simulink model "collision"  (R2018a)
settings: Solver=VariableStepAuto  StartTime=0.0  StopTime=120  FixedStep=0.01  MaxStep=.01  RelTol=1e-3
settings Model: Creator=U500304  LastModifiedBy=U500304
settings SolverCC: ZeroCrossAlgorithm=Adaptive
settings DataIOCC: SaveOutput=off  SaveTime=off
settings DebuggingCC: MaxConsecutiveZCsMsg=warning

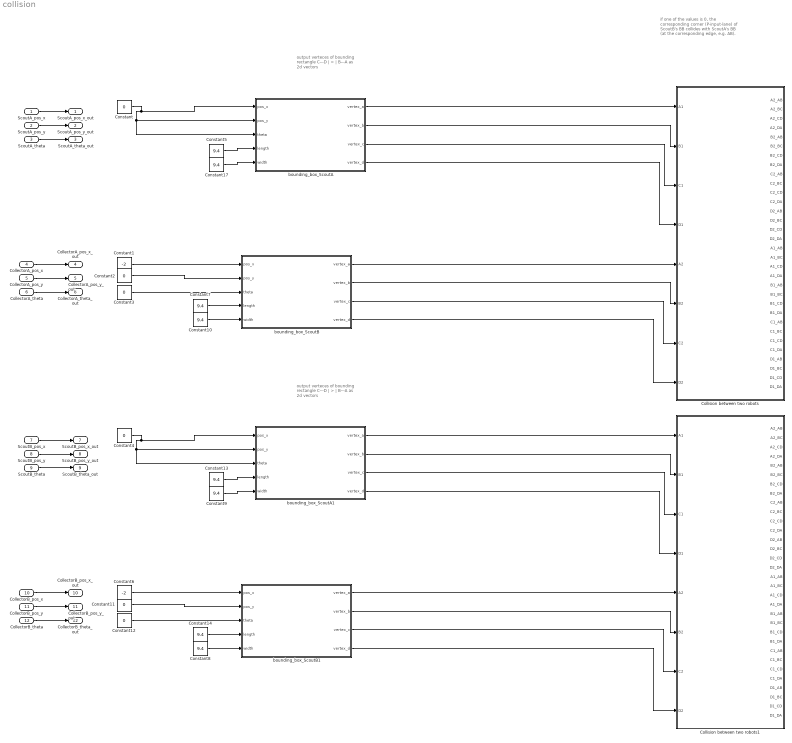
== system collision ==
  note: if one of the values is 0, the corresponding corner (P-input-lane) of ScoutB's BB collides with ScoutA's BB (at the corresponding edge, e.g. AB).
  note: output verteces of
      | bounding rectangle
      | C---D
      | |  >  |
      | B---A  as 2d vectors
  note: output verteces of
      | bounding rectangle
      | C---D
      | |  >  |
      | B---A  as 2d vectors
  ScoutA_pos_x : Inport  OutDataTypeStr=double  PortDimensions=1  SampleTime=0
  ScoutA_pos_y : Inport  Port=2  OutDataTypeStr=double  PortDimensions=1  SampleTime=0
  ScoutA_theta : Inport  Port=3  OutDataTypeStr=double  PortDimensions=1  SampleTime=0
  CollectorA_pos_x : Inport  Port=4  OutDataTypeStr=double  PortDimensions=1  SampleTime=0
  CollectorA_pos_y : Inport  Port=5  OutDataTypeStr=double  PortDimensions=1  SampleTime=0
  CollectorA_theta : Inport  Port=6  OutDataTypeStr=double  PortDimensions=1  SampleTime=0
  ScoutB_pos_x : Inport  Port=7  OutDataTypeStr=double  PortDimensions=1  SampleTime=0
  ScoutB_pos_y : Inport  Port=8  OutDataTypeStr=double  PortDimensions=1  SampleTime=0
  ScoutB_theta : Inport  Port=9  OutDataTypeStr=double  PortDimensions=1  SampleTime=0
  CollectorB_pos_x : Inport  Port=10  OutDataTypeStr=double  PortDimensions=1  SampleTime=0
  CollectorB_pos_y : Inport  Port=11  OutDataTypeStr=double  PortDimensions=1  SampleTime=0
  CollectorB_theta : Inport  Port=12  OutDataTypeStr=double  PortDimensions=1  SampleTime=0
  Collision between two robots : Subsystem
  Collision between two robots1 : Subsystem
  Constant{,2..4,11..12} (6 alike) : Constant  Value=0
  Constant1 : Constant  Value=-2
  Constant{5,7..10,13..14,17} (8 alike) : Constant  Value=9.4
  Constant6 : Constant  Value=-2
  bounding_box_ScoutA : Subsystem
  bounding_box_ScoutA1 : Subsystem
  bounding_box_ScoutB : Subsystem
  bounding_box_ScoutB1 : Subsystem
  ScoutA_pos_x_out : Outport
  ScoutA_pos_y_out : Outport  Port=2
  ScoutA_theta_out : Outport  Port=3
  CollectorA_pos_x_out : Outport  Port=4
  CollectorA_pos_y_out : Outport  Port=5
  CollectorA_theta_out : Outport  Port=6
  ScoutB_pos_x_out : Outport  Port=7
  ScoutB_pos_y_out : Outport  Port=8
  ScoutB_theta_out : Outport  Port=9
  CollectorB_pos_x_out : Outport  Port=10
  CollectorB_pos_y_out : Outport  Port=11
  CollectorB_theta_out : Outport  Port=12
  wires:
  Constant10/1 -> bounding_box_ScoutB/5(width)
  Constant17/1 -> bounding_box_ScoutA/5(width)
  Constant7/1 -> bounding_box_ScoutB/4(length)
  Constant3/1 -> bounding_box_ScoutB/3(theta)
  Constant5/1 -> bounding_box_ScoutA/4(length)
  Constant1/1 -> bounding_box_ScoutB/1(pos_x)
  Constant2/1 -> bounding_box_ScoutB/2(pos_y)
  Constant/1 -> bounding_box_ScoutA/3(theta), bounding_box_ScoutA/2(pos_y), bounding_box_ScoutA/1(pos_x)
  bounding_box_ScoutA/1(vertex_a) -> Collision between two robots/1(A1)
  bounding_box_ScoutA/2(vertex_b) -> Collision between two robots/2(B1)
  bounding_box_ScoutA/3(vertex_c) -> Collision between two robots/3(C1)
  bounding_box_ScoutA/4(vertex_d) -> Collision between two robots/4(D1)
  bounding_box_ScoutB/1(vertex_a) -> Collision between two robots/5(A2)
  bounding_box_ScoutB/2(vertex_b) -> Collision between two robots/6(B2)
  bounding_box_ScoutB/3(vertex_c) -> Collision between two robots/7(C2)
  bounding_box_ScoutB/4(vertex_d) -> Collision between two robots/8(D2)
  bounding_box_ScoutB1/4(vertex_d) -> Collision between two robots1/8(D2)
  bounding_box_ScoutB1/3(vertex_c) -> Collision between two robots1/7(C2)
  bounding_box_ScoutB1/2(vertex_b) -> Collision between two robots1/6(B2)
  bounding_box_ScoutB1/1(vertex_a) -> Collision between two robots1/5(A2)
  bounding_box_ScoutA1/4(vertex_d) -> Collision between two robots1/4(D1)
  bounding_box_ScoutA1/3(vertex_c) -> Collision between two robots1/3(C1)
  bounding_box_ScoutA1/2(vertex_b) -> Collision between two robots1/2(B1)
  bounding_box_ScoutA1/1(vertex_a) -> Collision between two robots1/1(A1)
  Constant4/1 -> bounding_box_ScoutA1/1(pos_x), bounding_box_ScoutA1/2(pos_y), bounding_box_ScoutA1/3(theta)
  Constant11/1 -> bounding_box_ScoutB1/2(pos_y)
  Constant6/1 -> bounding_box_ScoutB1/1(pos_x)
  Constant13/1 -> bounding_box_ScoutA1/4(length)
  Constant12/1 -> bounding_box_ScoutB1/3(theta)
  Constant14/1 -> bounding_box_ScoutB1/4(length)
  Constant9/1 -> bounding_box_ScoutA1/5(width)
  Constant8/1 -> bounding_box_ScoutB1/5(width)
  ScoutA_pos_x/1 -> ScoutA_pos_x_out/1
  ScoutA_pos_y/1 -> ScoutA_pos_y_out/1
  ScoutA_theta/1 -> ScoutA_theta_out/1
  CollectorA_pos_y/1 -> CollectorA_pos_y_out/1
  CollectorA_pos_x/1 -> CollectorA_pos_x_out/1
  CollectorA_theta/1 -> CollectorA_theta_out/1
  ScoutB_theta/1 -> ScoutB_theta_out/1
  ScoutB_pos_y/1 -> ScoutB_pos_y_out/1
  ScoutB_pos_x/1 -> ScoutB_pos_x_out/1
  CollectorB_theta/1 -> CollectorB_theta_out/1
  CollectorB_pos_y/1 -> CollectorB_pos_y_out/1
  CollectorB_pos_x/1 -> CollectorB_pos_x_out/1

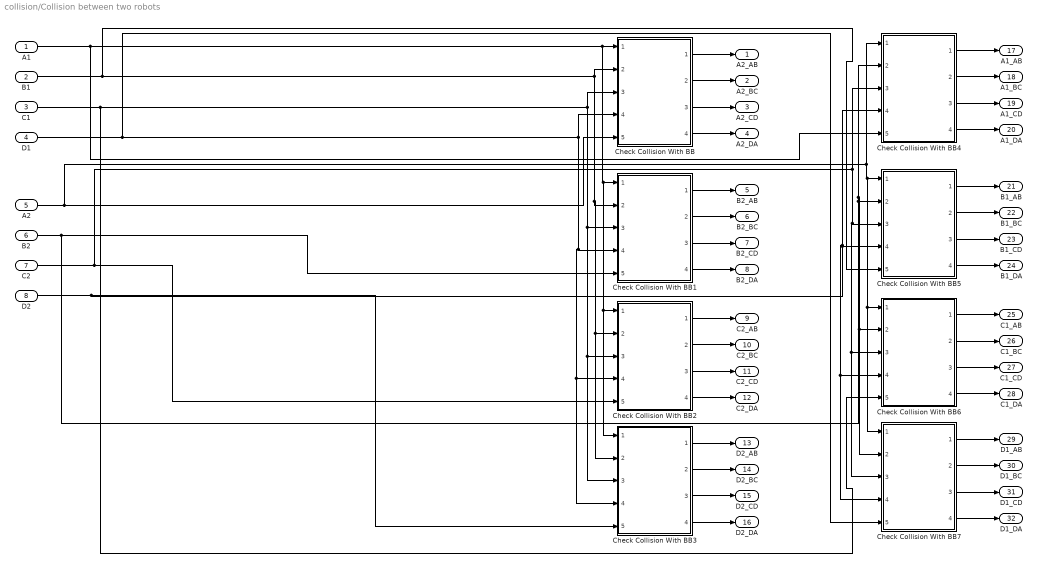
== system collision/Collision between two robots ==
  A1 : Inport
  B1 : Inport  Port=2
  C1 : Inport  Port=3
  D1 : Inport  Port=4
  A2 : Inport  Port=5
  B2 : Inport  Port=6
  C2 : Inport  Port=7
  D2 : Inport  Port=8
  Check Collision With BB{,1..7} (8 alike) : ModelReference  ModelNameDialog=check_collision_with_bounding  SimulationMode=Normal  ModelReferenceVersion=1.644
  A2_AB : Outport
  A2_BC : Outport  Port=2
  A2_CD : Outport  Port=3
  A2_DA : Outport  Port=4
  B2_AB : Outport  Port=5
  B2_BC : Outport  Port=6
  B2_CD : Outport  Port=7
  B2_DA : Outport  Port=8
  C2_AB : Outport  Port=9
  C2_BC : Outport  Port=10
  C2_CD : Outport  Port=11
  C2_DA : Outport  Port=12
  D2_AB : Outport  Port=13
  D2_BC : Outport  Port=14
  D2_CD : Outport  Port=15
  D2_DA : Outport  Port=16
  A1_AB : Outport  Port=17
  A1_BC : Outport  Port=18
  A1_CD : Outport  Port=19
  A1_DA : Outport  Port=20
  B1_AB : Outport  Port=21
  B1_BC : Outport  Port=22
  B1_CD : Outport  Port=23
  B1_DA : Outport  Port=24
  C1_AB : Outport  Port=25
  C1_BC : Outport  Port=26
  C1_CD : Outport  Port=27
  C1_DA : Outport  Port=28
  D1_AB : Outport  Port=29
  D1_BC : Outport  Port=30
  D1_CD : Outport  Port=31
  D1_DA : Outport  Port=32
  wires:
  Check Collision With BB3/3 -> D2_CD/1
  Check Collision With BB2/3 -> C2_CD/1
  Check Collision With BB/4 -> A2_DA/1
  Check Collision With BB/3 -> A2_CD/1
  Check Collision With BB1/3 -> B2_CD/1
  Check Collision With BB1/2 -> B2_BC/1
  Check Collision With BB2/1 -> C2_AB/1
  Check Collision With BB1/4 -> B2_DA/1
  Check Collision With BB/1 -> A2_AB/1
  Check Collision With BB1/1 -> B2_AB/1
  Check Collision With BB/2 -> A2_BC/1
  Check Collision With BB2/2 -> C2_BC/1
  Check Collision With BB3/4 -> D2_DA/1
  Check Collision With BB2/4 -> C2_DA/1
  Check Collision With BB3/1 -> D2_AB/1
  Check Collision With BB3/2 -> D2_BC/1
  Check Collision With BB6/3 -> C1_CD/1
  Check Collision With BB7/3 -> D1_CD/1
  Check Collision With BB7/1 -> D1_AB/1
  Check Collision With BB6/1 -> C1_AB/1
  Check Collision With BB7/4 -> D1_DA/1
  Check Collision With BB7/2 -> D1_BC/1
  Check Collision With BB4/4 -> A1_DA/1
  Check Collision With BB5/1 -> B1_AB/1
  Check Collision With BB5/4 -> B1_DA/1
  Check Collision With BB5/2 -> B1_BC/1
  Check Collision With BB4/3 -> A1_CD/1
  Check Collision With BB5/3 -> B1_CD/1
  D2/1 -> Check Collision With BB4/4, Check Collision With BB7/4, Check Collision With BB6/4, Check Collision With BB5/4, Check Collision With BB3/5
  Check Collision With BB4/1 -> A1_AB/1
  B2/1 -> Check Collision With BB4/2, Check Collision With BB7/2, Check Collision With BB6/2, Check Collision With BB5/2, Check Collision With BB1/5
  B1/1 -> Check Collision With BB5/5, Check Collision With BB/2, Check Collision With BB3/2, Check Collision With BB2/2, Check Collision With BB1/2
  C1/1 -> Check Collision With BB6/5, Check Collision With BB/3, Check Collision With BB3/3, Check Collision With BB2/3, Check Collision With BB1/3
  D1/1 -> Check Collision With BB7/5, Check Collision With BB/4, Check Collision With BB3/4, Check Collision With BB2/4, Check Collision With BB1/4
  C2/1 -> Check Collision With BB4/3, Check Collision With BB7/3, Check Collision With BB6/3, Check Collision With BB5/3, Check Collision With BB2/5
  Check Collision With BB6/2 -> C1_BC/1
  A2/1 -> Check Collision With BB4/1, Check Collision With BB7/1, Check Collision With BB6/1, Check Collision With BB5/1, Check Collision With BB/5
  Check Collision With BB4/2 -> A1_BC/1
  A1/1 -> Check Collision With BB4/5, Check Collision With BB/1, Check Collision With BB3/1, Check Collision With BB2/1, Check Collision With BB1/1
  Check Collision With BB6/4 -> C1_DA/1

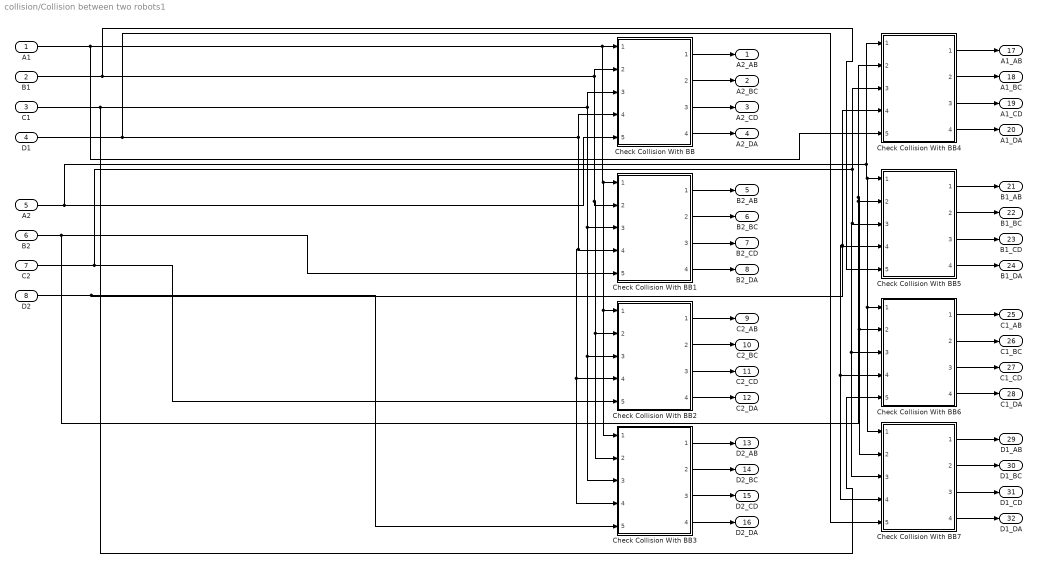
== system collision/Collision between two robots1 ==
  A1 : Inport
  B1 : Inport  Port=2
  C1 : Inport  Port=3
  D1 : Inport  Port=4
  A2 : Inport  Port=5
  B2 : Inport  Port=6
  C2 : Inport  Port=7
  D2 : Inport  Port=8
  Check Collision With BB{,1..7} (8 alike) : ModelReference  ModelNameDialog=check_collision_with_bounding  SimulationMode=Normal  ModelReferenceVersion=1.644
  A2_AB : Outport
  A2_BC : Outport  Port=2
  A2_CD : Outport  Port=3
  A2_DA : Outport  Port=4
  B2_AB : Outport  Port=5
  B2_BC : Outport  Port=6
  B2_CD : Outport  Port=7
  B2_DA : Outport  Port=8
  C2_AB : Outport  Port=9
  C2_BC : Outport  Port=10
  C2_CD : Outport  Port=11
  C2_DA : Outport  Port=12
  D2_AB : Outport  Port=13
  D2_BC : Outport  Port=14
  D2_CD : Outport  Port=15
  D2_DA : Outport  Port=16
  A1_AB : Outport  Port=17
  A1_BC : Outport  Port=18
  A1_CD : Outport  Port=19
  A1_DA : Outport  Port=20
  B1_AB : Outport  Port=21
  B1_BC : Outport  Port=22
  B1_CD : Outport  Port=23
  B1_DA : Outport  Port=24
  C1_AB : Outport  Port=25
  C1_BC : Outport  Port=26
  C1_CD : Outport  Port=27
  C1_DA : Outport  Port=28
  D1_AB : Outport  Port=29
  D1_BC : Outport  Port=30
  D1_CD : Outport  Port=31
  D1_DA : Outport  Port=32
  wires:
  Check Collision With BB6/4 -> C1_DA/1
  A1/1 -> Check Collision With BB1/1, Check Collision With BB2/1, Check Collision With BB3/1, Check Collision With BB/1, Check Collision With BB4/5
  Check Collision With BB4/2 -> A1_BC/1
  A2/1 -> Check Collision With BB/5, Check Collision With BB5/1, Check Collision With BB6/1, Check Collision With BB7/1, Check Collision With BB4/1
  Check Collision With BB6/2 -> C1_BC/1
  C2/1 -> Check Collision With BB2/5, Check Collision With BB5/3, Check Collision With BB6/3, Check Collision With BB7/3, Check Collision With BB4/3
  D1/1 -> Check Collision With BB1/4, Check Collision With BB2/4, Check Collision With BB3/4, Check Collision With BB/4, Check Collision With BB7/5
  C1/1 -> Check Collision With BB1/3, Check Collision With BB2/3, Check Collision With BB3/3, Check Collision With BB/3, Check Collision With BB6/5
  B1/1 -> Check Collision With BB1/2, Check Collision With BB2/2, Check Collision With BB3/2, Check Collision With BB/2, Check Collision With BB5/5
  B2/1 -> Check Collision With BB1/5, Check Collision With BB5/2, Check Collision With BB6/2, Check Collision With BB7/2, Check Collision With BB4/2
  Check Collision With BB4/1 -> A1_AB/1
  D2/1 -> Check Collision With BB3/5, Check Collision With BB5/4, Check Collision With BB6/4, Check Collision With BB7/4, Check Collision With BB4/4
  Check Collision With BB5/3 -> B1_CD/1
  Check Collision With BB4/3 -> A1_CD/1
  Check Collision With BB5/2 -> B1_BC/1
  Check Collision With BB5/4 -> B1_DA/1
  Check Collision With BB5/1 -> B1_AB/1
  Check Collision With BB4/4 -> A1_DA/1
  Check Collision With BB7/2 -> D1_BC/1
  Check Collision With BB7/4 -> D1_DA/1
  Check Collision With BB6/1 -> C1_AB/1
  Check Collision With BB7/1 -> D1_AB/1
  Check Collision With BB7/3 -> D1_CD/1
  Check Collision With BB6/3 -> C1_CD/1
  Check Collision With BB3/2 -> D2_BC/1
  Check Collision With BB3/1 -> D2_AB/1
  Check Collision With BB2/4 -> C2_DA/1
  Check Collision With BB3/4 -> D2_DA/1
  Check Collision With BB2/2 -> C2_BC/1
  Check Collision With BB/2 -> A2_BC/1
  Check Collision With BB1/1 -> B2_AB/1
  Check Collision With BB/1 -> A2_AB/1
  Check Collision With BB1/4 -> B2_DA/1
  Check Collision With BB2/1 -> C2_AB/1
  Check Collision With BB1/2 -> B2_BC/1
  Check Collision With BB1/3 -> B2_CD/1
  Check Collision With BB/3 -> A2_CD/1
  Check Collision With BB/4 -> A2_DA/1
  Check Collision With BB2/3 -> C2_CD/1
  Check Collision With BB3/3 -> D2_CD/1

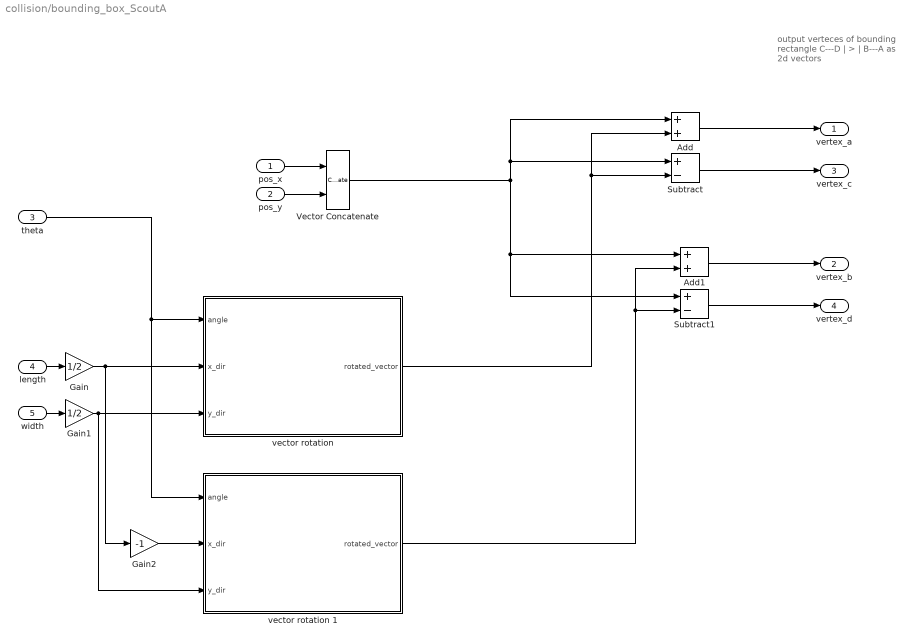
== system collision/bounding_box_ScoutA ==
  note: output verteces of
      | bounding rectangle
      | C---D
      | |  >  |
      | B---A  as 2d vectors
  pos_x : Inport
  pos_y : Inport  Port=2
  theta : Inport  Port=3
  length : Inport  Port=4
  width : Inport  Port=5
  Add : Sum
  Add1 : Sum
  Gain : Gain  Gain=1/2
  Gain1 : Gain  Gain=1/2
  Gain2 : Gain  Gain=-1
  Subtract : Sum  Inputs=+-
  Subtract1 : Sum  Inputs=+-
  Vector Concatenate : Concatenate
  "vector rotation " : Subsystem
  vector rotation 1 : Subsystem
  vertex_a : Outport
  vertex_b : Outport  Port=2
  vertex_c : Outport  Port=3
  vertex_d : Outport  Port=4
  wires:
  width/1 -> Gain1/1
  length/1 -> Gain/1
  pos_x/1 -> Vector Concatenate/1
  pos_y/1 -> Vector Concatenate/2
  theta/1 -> vector rotation 1/1(angle), "vector rotation "/1(angle)
  Gain/1 -> Gain2/1, "vector rotation "/2(x_dir)
  Gain2/1 -> vector rotation 1/2(x_dir)
  Gain1/1 -> vector rotation 1/3(y_dir), "vector rotation "/3(y_dir)
  Vector Concatenate/1 -> Subtract1/1, Add1/1, Subtract/1, Add/1
  "vector rotation "/1("rotated_vector ") -> Subtract/2, Add/2
  vector rotation 1/1("rotated_vector ") -> Subtract1/2, Add1/2
  Add/1 -> vertex_a/1
  Subtract/1 -> vertex_c/1
  Add1/1 -> vertex_b/1
  Subtract1/1 -> vertex_d/1

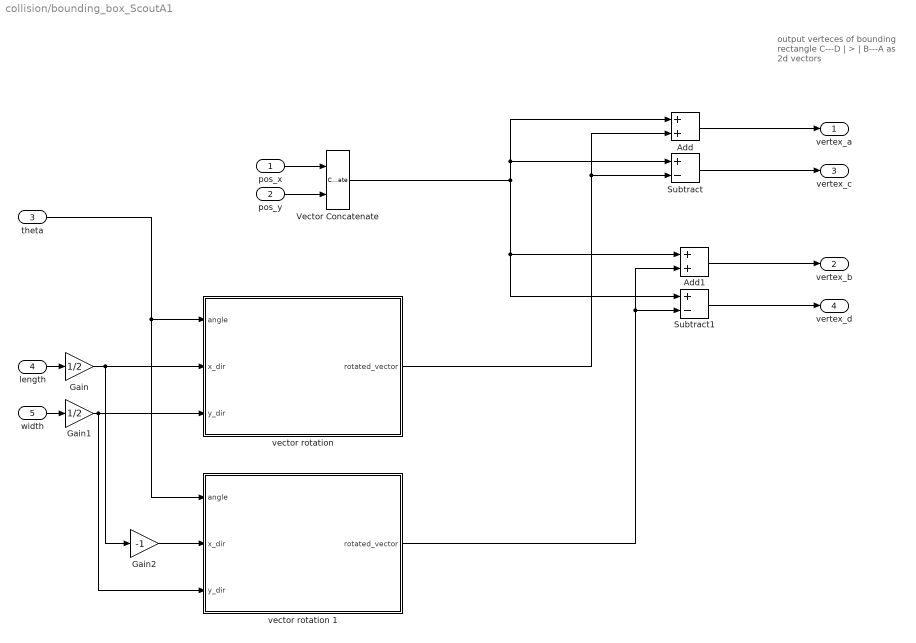
== system collision/bounding_box_ScoutA1 ==
  note: output verteces of
      | bounding rectangle
      | C---D
      | |  >  |
      | B---A  as 2d vectors
  pos_x : Inport
  pos_y : Inport  Port=2
  theta : Inport  Port=3
  length : Inport  Port=4
  width : Inport  Port=5
  Add : Sum
  Add1 : Sum
  Gain : Gain  Gain=1/2
  Gain1 : Gain  Gain=1/2
  Gain2 : Gain  Gain=-1
  Subtract : Sum  Inputs=+-
  Subtract1 : Sum  Inputs=+-
  Vector Concatenate : Concatenate
  "vector rotation " : Subsystem
  vector rotation 1 : Subsystem
  vertex_a : Outport
  vertex_b : Outport  Port=2
  vertex_c : Outport  Port=3
  vertex_d : Outport  Port=4
  wires:
  Subtract1/1 -> vertex_d/1
  Add1/1 -> vertex_b/1
  Subtract/1 -> vertex_c/1
  Add/1 -> vertex_a/1
  vector rotation 1/1("rotated_vector ") -> Add1/2, Subtract1/2
  "vector rotation "/1("rotated_vector ") -> Add/2, Subtract/2
  Vector Concatenate/1 -> Add/1, Subtract/1, Add1/1, Subtract1/1
  Gain1/1 -> "vector rotation "/3(y_dir), vector rotation 1/3(y_dir)
  Gain2/1 -> vector rotation 1/2(x_dir)
  Gain/1 -> "vector rotation "/2(x_dir), Gain2/1
  theta/1 -> "vector rotation "/1(angle), vector rotation 1/1(angle)
  pos_y/1 -> Vector Concatenate/2
  pos_x/1 -> Vector Concatenate/1
  length/1 -> Gain/1
  width/1 -> Gain1/1

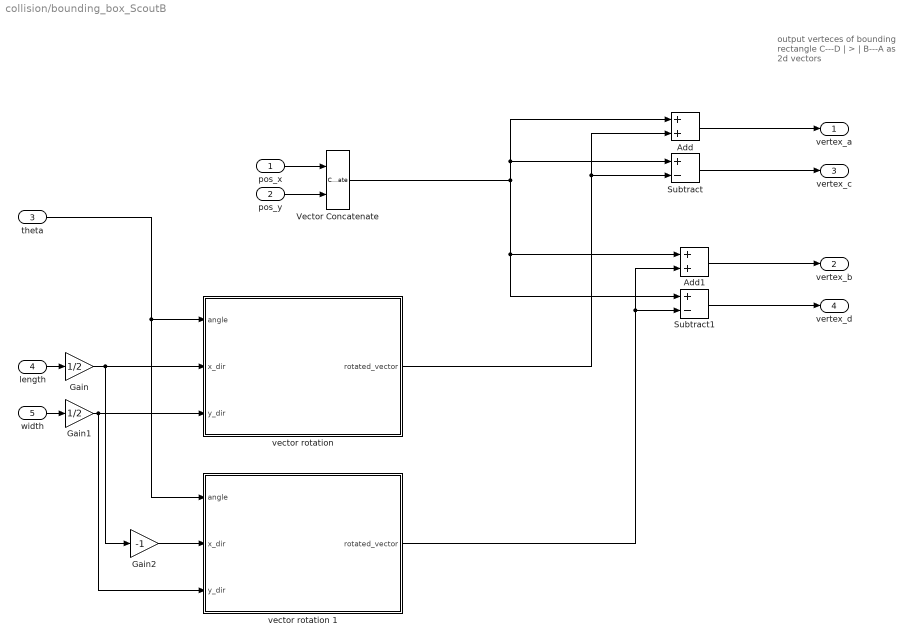
== system collision/bounding_box_ScoutB ==
  note: output verteces of
      | bounding rectangle
      | C---D
      | |  >  |
      | B---A  as 2d vectors
  pos_x : Inport
  pos_y : Inport  Port=2
  theta : Inport  Port=3
  length : Inport  Port=4
  width : Inport  Port=5
  Add : Sum
  Add1 : Sum
  Gain : Gain  Gain=1/2
  Gain1 : Gain  Gain=1/2
  Gain2 : Gain  Gain=-1
  Subtract : Sum  Inputs=+-
  Subtract1 : Sum  Inputs=+-
  Vector Concatenate : Concatenate
  "vector rotation " : Subsystem
  vector rotation 1 : Subsystem
  vertex_a : Outport
  vertex_b : Outport  Port=2
  vertex_c : Outport  Port=3
  vertex_d : Outport  Port=4
  wires:
  width/1 -> Gain1/1
  length/1 -> Gain/1
  pos_x/1 -> Vector Concatenate/1
  pos_y/1 -> Vector Concatenate/2
  theta/1 -> vector rotation 1/1(angle), "vector rotation "/1(angle)
  Gain/1 -> Gain2/1, "vector rotation "/2(x_dir)
  Gain2/1 -> vector rotation 1/2(x_dir)
  Gain1/1 -> vector rotation 1/3(y_dir), "vector rotation "/3(y_dir)
  Vector Concatenate/1 -> Subtract1/1, Add1/1, Subtract/1, Add/1
  "vector rotation "/1("rotated_vector ") -> Subtract/2, Add/2
  vector rotation 1/1("rotated_vector ") -> Subtract1/2, Add1/2
  Add/1 -> vertex_a/1
  Subtract/1 -> vertex_c/1
  Add1/1 -> vertex_b/1
  Subtract1/1 -> vertex_d/1

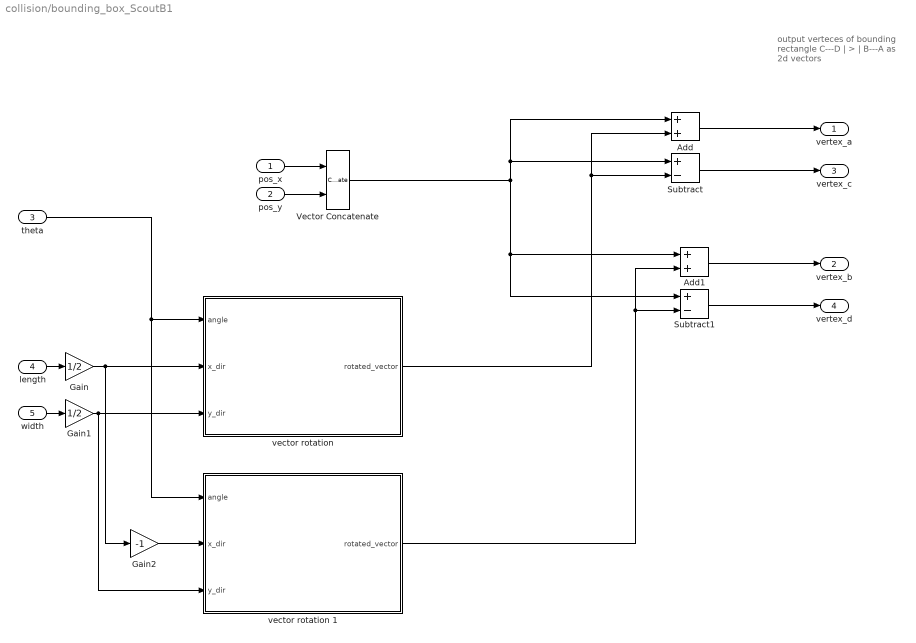
== system collision/bounding_box_ScoutB1 ==
  note: output verteces of
      | bounding rectangle
      | C---D
      | |  >  |
      | B---A  as 2d vectors
  pos_x : Inport
  pos_y : Inport  Port=2
  theta : Inport  Port=3
  length : Inport  Port=4
  width : Inport  Port=5
  Add : Sum
  Add1 : Sum
  Gain : Gain  Gain=1/2
  Gain1 : Gain  Gain=1/2
  Gain2 : Gain  Gain=-1
  Subtract : Sum  Inputs=+-
  Subtract1 : Sum  Inputs=+-
  Vector Concatenate : Concatenate
  "vector rotation " : Subsystem
  vector rotation 1 : Subsystem
  vertex_a : Outport
  vertex_b : Outport  Port=2
  vertex_c : Outport  Port=3
  vertex_d : Outport  Port=4
  wires:
  Subtract1/1 -> vertex_d/1
  Add1/1 -> vertex_b/1
  Subtract/1 -> vertex_c/1
  Add/1 -> vertex_a/1
  vector rotation 1/1("rotated_vector ") -> Add1/2, Subtract1/2
  "vector rotation "/1("rotated_vector ") -> Add/2, Subtract/2
  Vector Concatenate/1 -> Add/1, Subtract/1, Add1/1, Subtract1/1
  Gain1/1 -> "vector rotation "/3(y_dir), vector rotation 1/3(y_dir)
  Gain2/1 -> vector rotation 1/2(x_dir)
  Gain/1 -> "vector rotation "/2(x_dir), Gain2/1
  theta/1 -> "vector rotation "/1(angle), vector rotation 1/1(angle)
  pos_y/1 -> Vector Concatenate/2
  pos_x/1 -> Vector Concatenate/1
  length/1 -> Gain/1
  width/1 -> Gain1/1

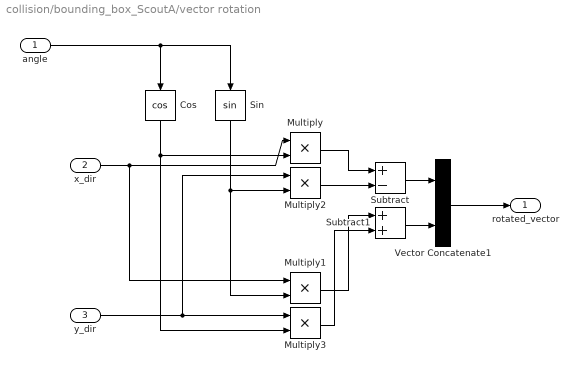
== system collision/bounding_box_ScoutA/vector rotation  ==
  angle : Inport
  x_dir : Inport  Port=2
  y_dir : Inport  Port=3
  Cos : Trigonometry  Operator=cos
  Multiply{,1..3} (4 alike) : Product
  Sin : Trigonometry
  Subtract : Sum  Inputs=+-
  Subtract1 : Sum
  Vector Concatenate1 : Concatenate
  "rotated_vector " : Outport
  wires:
  Multiply3/1 -> Subtract1/2
  Multiply1/1 -> Subtract1/1
  Multiply/1 -> Subtract/1
  y_dir/1 -> Multiply3/1, Multiply2/1
  Subtract1/1 -> Vector Concatenate1/2
  Cos/1 -> Multiply3/2, Multiply/2
  Sin/1 -> Multiply1/2, Multiply2/2
  angle/1 -> Cos/1, Sin/1
  x_dir/1 -> Multiply1/1, Multiply/1
  Vector Concatenate1/1 -> "rotated_vector "/1
  Subtract/1 -> Vector Concatenate1/1
  Multiply2/1 -> Subtract/2

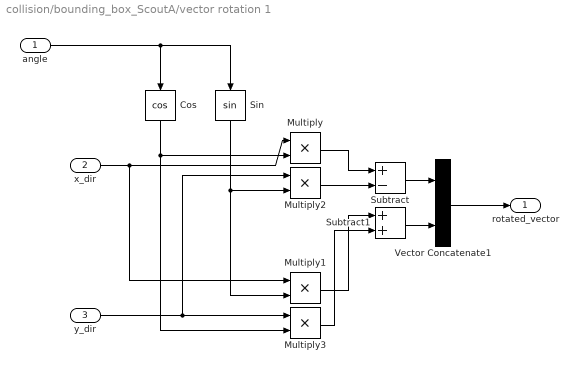
== system collision/bounding_box_ScoutA/vector rotation 1 ==
  angle : Inport
  x_dir : Inport  Port=2
  y_dir : Inport  Port=3
  Cos : Trigonometry  Operator=cos
  Multiply{,1..3} (4 alike) : Product
  Sin : Trigonometry
  Subtract : Sum  Inputs=+-
  Subtract1 : Sum
  Vector Concatenate1 : Concatenate
  "rotated_vector " : Outport
  wires:
  Multiply2/1 -> Subtract/2
  Subtract/1 -> Vector Concatenate1/1
  Vector Concatenate1/1 -> "rotated_vector "/1
  x_dir/1 -> Multiply/1, Multiply1/1
  angle/1 -> Sin/1, Cos/1
  Sin/1 -> Multiply2/2, Multiply1/2
  Cos/1 -> Multiply/2, Multiply3/2
  Subtract1/1 -> Vector Concatenate1/2
  y_dir/1 -> Multiply2/1, Multiply3/1
  Multiply/1 -> Subtract/1
  Multiply1/1 -> Subtract1/1
  Multiply3/1 -> Subtract1/2

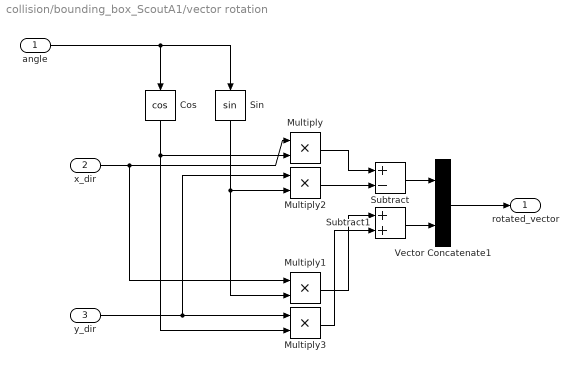
== system collision/bounding_box_ScoutA1/vector rotation  ==
  angle : Inport
  x_dir : Inport  Port=2
  y_dir : Inport  Port=3
  Cos : Trigonometry  Operator=cos
  Multiply{,1..3} (4 alike) : Product
  Sin : Trigonometry
  Subtract : Sum  Inputs=+-
  Subtract1 : Sum
  Vector Concatenate1 : Concatenate
  "rotated_vector " : Outport
  wires:
  Multiply2/1 -> Subtract/2
  Subtract/1 -> Vector Concatenate1/1
  Vector Concatenate1/1 -> "rotated_vector "/1
  x_dir/1 -> Multiply/1, Multiply1/1
  angle/1 -> Sin/1, Cos/1
  Sin/1 -> Multiply2/2, Multiply1/2
  Cos/1 -> Multiply/2, Multiply3/2
  Subtract1/1 -> Vector Concatenate1/2
  y_dir/1 -> Multiply2/1, Multiply3/1
  Multiply/1 -> Subtract/1
  Multiply1/1 -> Subtract1/1
  Multiply3/1 -> Subtract1/2

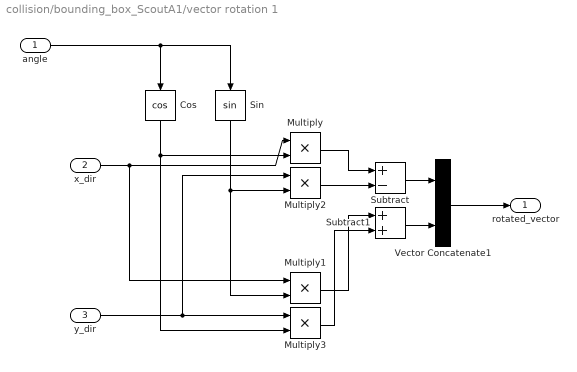
== system collision/bounding_box_ScoutA1/vector rotation 1 ==
  angle : Inport
  x_dir : Inport  Port=2
  y_dir : Inport  Port=3
  Cos : Trigonometry  Operator=cos
  Multiply{,1..3} (4 alike) : Product
  Sin : Trigonometry
  Subtract : Sum  Inputs=+-
  Subtract1 : Sum
  Vector Concatenate1 : Concatenate
  "rotated_vector " : Outport
  wires:
  Multiply3/1 -> Subtract1/2
  Multiply1/1 -> Subtract1/1
  Multiply/1 -> Subtract/1
  y_dir/1 -> Multiply3/1, Multiply2/1
  Subtract1/1 -> Vector Concatenate1/2
  Cos/1 -> Multiply3/2, Multiply/2
  Sin/1 -> Multiply1/2, Multiply2/2
  angle/1 -> Cos/1, Sin/1
  x_dir/1 -> Multiply1/1, Multiply/1
  Vector Concatenate1/1 -> "rotated_vector "/1
  Subtract/1 -> Vector Concatenate1/1
  Multiply2/1 -> Subtract/2

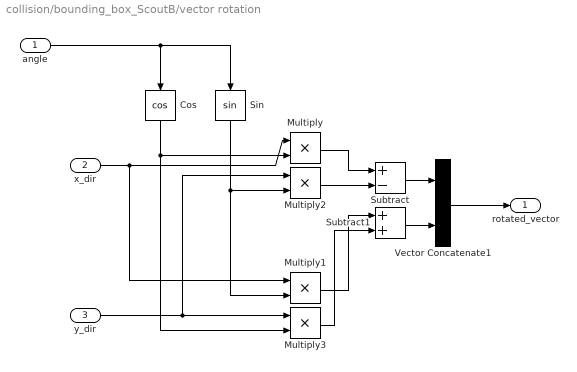
== system collision/bounding_box_ScoutB/vector rotation  ==
  angle : Inport
  x_dir : Inport  Port=2
  y_dir : Inport  Port=3
  Cos : Trigonometry  Operator=cos
  Multiply{,1..3} (4 alike) : Product
  Sin : Trigonometry
  Subtract : Sum  Inputs=+-
  Subtract1 : Sum
  Vector Concatenate1 : Concatenate
  "rotated_vector " : Outport
  wires:
  Multiply3/1 -> Subtract1/2
  Multiply1/1 -> Subtract1/1
  Multiply/1 -> Subtract/1
  y_dir/1 -> Multiply3/1, Multiply2/1
  Subtract1/1 -> Vector Concatenate1/2
  Cos/1 -> Multiply3/2, Multiply/2
  Sin/1 -> Multiply1/2, Multiply2/2
  angle/1 -> Cos/1, Sin/1
  x_dir/1 -> Multiply1/1, Multiply/1
  Vector Concatenate1/1 -> "rotated_vector "/1
  Subtract/1 -> Vector Concatenate1/1
  Multiply2/1 -> Subtract/2

== system collision/bounding_box_ScoutB/vector rotation 1 ==
  angle : Inport
  x_dir : Inport  Port=2
  y_dir : Inport  Port=3
  Cos : Trigonometry  Operator=cos
  Multiply{,1..3} (4 alike) : Product
  Sin : Trigonometry
  Subtract : Sum  Inputs=+-
  Subtract1 : Sum
  Vector Concatenate1 : Concatenate
  "rotated_vector " : Outport
  wires:
  Multiply2/1 -> Subtract/2
  Subtract/1 -> Vector Concatenate1/1
  Vector Concatenate1/1 -> "rotated_vector "/1
  x_dir/1 -> Multiply/1, Multiply1/1
  angle/1 -> Sin/1, Cos/1
  Sin/1 -> Multiply2/2, Multiply1/2
  Cos/1 -> Multiply/2, Multiply3/2
  Subtract1/1 -> Vector Concatenate1/2
  y_dir/1 -> Multiply2/1, Multiply3/1
  Multiply/1 -> Subtract/1
  Multiply1/1 -> Subtract1/1
  Multiply3/1 -> Subtract1/2

== system collision/bounding_box_ScoutB1/vector rotation  ==
  angle : Inport
  x_dir : Inport  Port=2
  y_dir : Inport  Port=3
  Cos : Trigonometry  Operator=cos
  Multiply{,1..3} (4 alike) : Product
  Sin : Trigonometry
  Subtract : Sum  Inputs=+-
  Subtract1 : Sum
  Vector Concatenate1 : Concatenate
  "rotated_vector " : Outport
  wires:
  Multiply2/1 -> Subtract/2
  Subtract/1 -> Vector Concatenate1/1
  Vector Concatenate1/1 -> "rotated_vector "/1
  x_dir/1 -> Multiply/1, Multiply1/1
  angle/1 -> Sin/1, Cos/1
  Sin/1 -> Multiply2/2, Multiply1/2
  Cos/1 -> Multiply/2, Multiply3/2
  Subtract1/1 -> Vector Concatenate1/2
  y_dir/1 -> Multiply2/1, Multiply3/1
  Multiply/1 -> Subtract/1
  Multiply1/1 -> Subtract1/1
  Multiply3/1 -> Subtract1/2

== system collision/bounding_box_ScoutB1/vector rotation 1 ==
  angle : Inport
  x_dir : Inport  Port=2
  y_dir : Inport  Port=3
  Cos : Trigonometry  Operator=cos
  Multiply{,1..3} (4 alike) : Product
  Sin : Trigonometry
  Subtract : Sum  Inputs=+-
  Subtract1 : Sum
  Vector Concatenate1 : Concatenate
  "rotated_vector " : Outport
  wires:
  Multiply3/1 -> Subtract1/2
  Multiply1/1 -> Subtract1/1
  Multiply/1 -> Subtract/1
  y_dir/1 -> Multiply3/1, Multiply2/1
  Subtract1/1 -> Vector Concatenate1/2
  Cos/1 -> Multiply3/2, Multiply/2
  Sin/1 -> Multiply1/2, Multiply2/2
  angle/1 -> Cos/1, Sin/1
  x_dir/1 -> Multiply1/1, Multiply/1
  Vector Concatenate1/1 -> "rotated_vector "/1
  Subtract/1 -> Vector Concatenate1/1
  Multiply2/1 -> Subtract/2
